simulink model "model_03_discrete"  (R2024b)
settings: Solver=FixedStepDiscrete  StartTime=0.0  StopTime=10.0  FixedStep=0.1  RelTol=1e-3
model workspace (MAT data in the model file):
  Kp = 3
  Ts = 0.1
  dend = [1 -1.5629 0.5629]
  numd = [0 0.3567 0.2946]
settings Model: Creator=santi  LastModifiedBy=santi

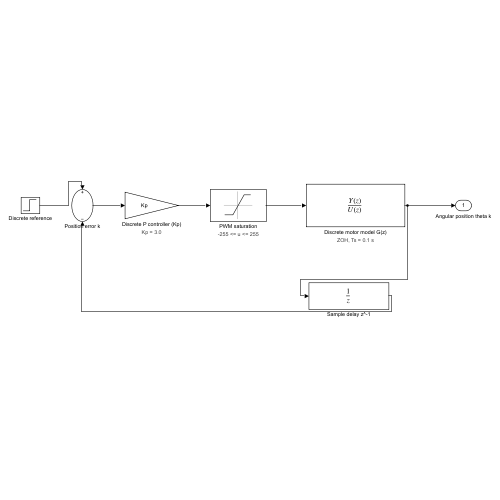
[thumbnail: Simulink's stored preview of the top-level diagram]
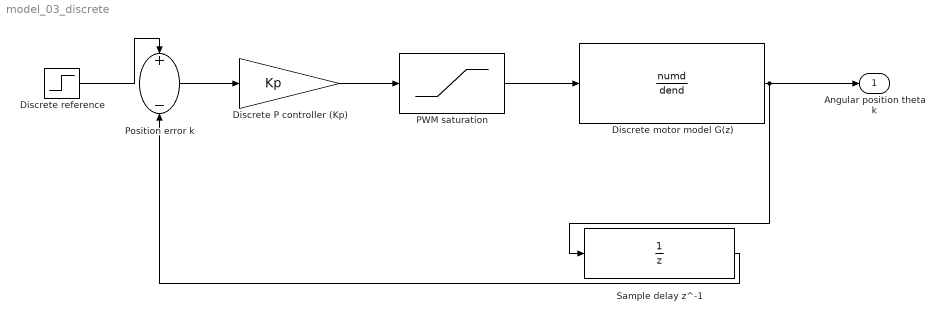
== system model_03_discrete ==
  Discrete P controller (Kp) : Gain  Gain=Kp  SampleTime=0.1
      settings: AttributesFormatString=Kp = 3.0
  Discrete motor model G(z) : DiscreteTransferFcn  Numerator=numd  Denominator=dend  SampleTime=Ts
      settings: AttributesFormatString=ZOH, Ts = 0.1 s
  Discrete reference : Step  After=45  SampleTime=0.1
  PWM saturation : Saturate  UpperLimit=255  LowerLimit=-255
      settings: AttributesFormatString=-255 <= u <= 255
  Position error k : Sum  Inputs=+-
  Sample delay z^-1 : UnitDelay  SampleTime=Ts  HasFrameUpgradeWarning=on
  Angular position theta k : Outport
  wires:
  Discrete reference/1 -> Position error k/1
  Position error k/1 -> Discrete P controller (Kp)/1
  Discrete P controller (Kp)/1 -> PWM saturation/1
  PWM saturation/1 -> Discrete motor model G(z)/1
  Discrete motor model G(z)/1 -> Angular position theta k/1, Sample delay z^-1/1
  Sample delay z^-1/1 -> Position error k/2
